simulink model "B34SNSTest"  (R2023b)
settings: Solver=VariableStepAuto  StartTime=0.0  StopTime=100  RelTol=1E-4  AbsTol=1E-4
values from neighbouring files (symbols this model uses):
  AinfKA_h_B34 = -60    [B34.m]    (also in CtrlParaSNSTuning.m)
  AinfKA_p_B34 = 1.0    (= 1)    [B34.m]    (also in CtrlParaSNSTuning.m)
  AinfKA_s_B34 = 1.0    (= 1)    [B34.m]    (also in CtrlParaSNSTuning.m)
  AKA_B34_0 = 0.4    [B34.m]    (also in CtrlParaSNSTuning.m; InitPara.m)
  BinfKA_h_B34 = -55.0    (= -55)    [B34.m]    (also in CtrlParaSNSTuning.m)
  BinfKA_p_B34 = 2.0    (= 2)    [B34.m]    (also in CtrlParaSNSTuning.m)
  BinfKA_s_B34 = 1.0    (= 1)    [B34.m]    (also in CtrlParaSNSTuning.m)
  BKA_B34_0 = 0.4    [B34.m]    (also in CtrlParaSNSTuning.m; InitPara.m)
  Cm_B34 = 0.01    [B34.m]    (also in CtrlParaSNSTuning.m)
  EKA_B34 = -60    [B34.m]    (also in CtrlParaSNSTuning.m)
  EL_B34 = -60    [B34.m]    (also in CtrlParaSNSTuning.m)
  gKA_B34 = 1.25    [B34.m]    (also in CtrlParaSNSTuning.m)
  gL_B34 = 0.1    [B34.m]    (also in CtrlParaSNSTuning.m)
  pKA_B34 = 2    [B34.m]    (also in CtrlParaSNSTuning.m)
  RKA_B34 = 0    [B34.m]    (also in CtrlParaSNSTuning.m)
  RL_B34 = 0    [B34.m]    (also in CtrlParaSNSTuning.m)
  tAKA_h_B34 = -56    [B34.m]    (also in CtrlParaSNSTuning.m)
  tAKA_p_B34 = 2.0    (= 2)    [B34.m]    (also in CtrlParaSNSTuning.m)
  tAKA_s_B34 = 1.0    (= 1)    [B34.m]    (also in CtrlParaSNSTuning.m)
  tAKA_tmax_B34 = 0.2    [B34.m]    (also in CtrlParaSNSTuning.m)
  tAKA_tmin_B34 = 0.02    [B34.m]    (also in CtrlParaSNSTuning.m)
  tBKA_tmax_B34 = 0.5    [B34.m]    (also in CtrlParaSNSTuning.m)
  V_B34_0 = -60    [B34.m]    (also in CtrlParaSNSTuning.m; InitPara.m)
  V_max = 130/3    (= 43.3333333333)    [B34.m]    (also in B4.m; CtrlParaSNSTuning.m)
  V_min = 3.2/3    (= 1.06666666667)    [B34.m]    (also in B4.m = 5; CtrlParaSNSTuning.m = 5)
undefined symbols (not defined in the file or in its folder): Iapp
settings Model: SimulationMode=accelerator  Creator=liyan  LastModifiedBy=Yanjun
settings ModelReferenceCC: EnableRefExpFcnMdlSchedulingChecks=on

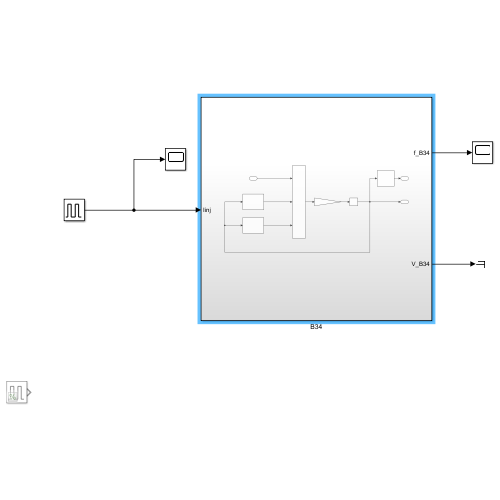
[thumbnail: Simulink's stored preview of the top-level diagram]
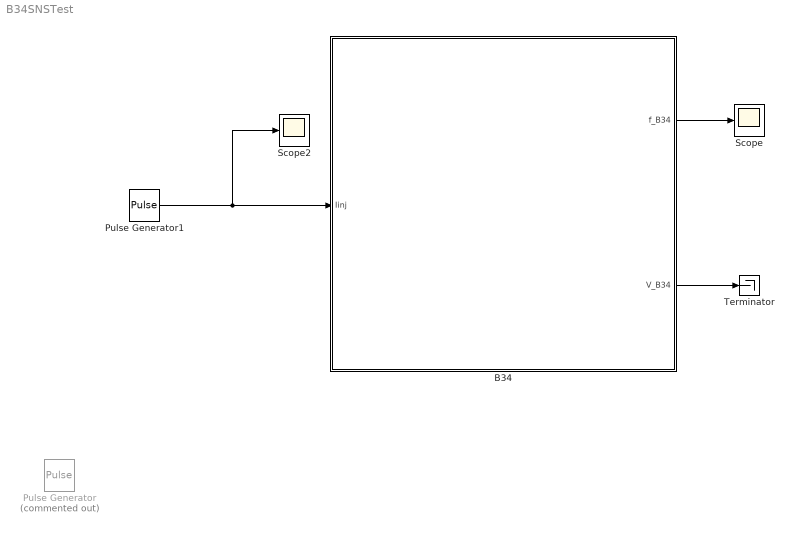
== system B34SNSTest ==
  B34 : Subsystem
      settings: PortSchema="{\"entries\":[{\"content\":{\"sides\":[{\"content\":{\"connectorIds\":[]},\"type\":\"ConnectorPlacement.EquallySpacedRectSide\",\"uuid\":\"791cb9f9-6115-440d-b81f-06b3e1381d11\"},{\"content\":{\"connectorIds\":[],\"side\":\"RIGHT\"},\"type\":\"ConnectorPlacement.EquallySpacedRectSide\",\"uuid\":\"7c3ff3b3-a19c-4513-b6da-d54d5819647a\"},{\"content\":{\"connectorIds\":[\"Out1\",\"Out2\"],\"side\":\"TOP\"},\"type\":\"ConnectorPlacement.EquallySpacedRectSide\",\"uuid\":\"74d2471c-8ad6-4c64-9275-9831c9b942a4\"},{\"content\":{\"connectorIds\":[\"In1\"],\"side\":\"BOTTOM\"},\"type\":\"ConnectorPlacement.EquallySpacedRectSide\",\"uuid\":\"d13eda8e-856d-496c-9126-6826d7a5e8e6\"}]},\"type\":\"ConnectorPlacement.EquallySpacedConnector\",\"uuid\":\"cfc5e95a-0097-4eeb-afba-0bc23a3dc93b\"}],\"packageUris\":[\"http://schema.mathworks.com/mf0/Connector/R2020b\"],\"version\":\"1.0\"}"
  Pulse Generator : DiscretePulseGenerator  Commented=on  PulseType=Time based  Amplitude=Iapp  Period=30  PulseWidth=10/30*100  PhaseDelay=10
  Pulse Generator1 : DiscretePulseGenerator  PulseType=Time based  Amplitude=Iapp  Period=100  PulseWidth=10/100*100  PhaseDelay=35
  Scope : Scope
  Scope2 : Scope
  Terminator : Terminator
  wires:
  Pulse Generator1/1 -> B34/1(Iinj), Scope2/1
  B34/2(f_B34) -> Scope/1
  B34/1(V_B34) -> Terminator/1

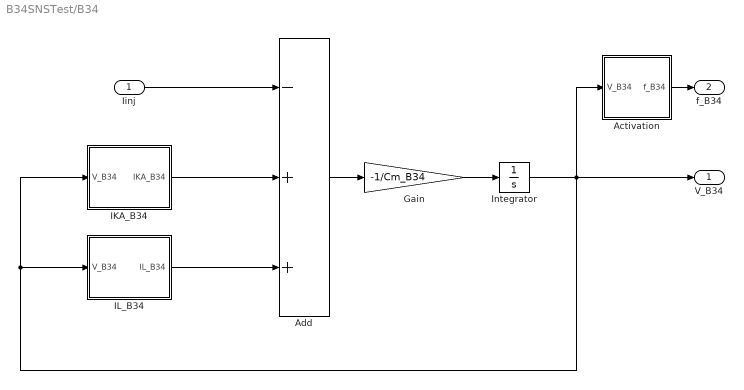
== system B34SNSTest/B34 ==
  Iinj : Inport
  Activation : Subsystem
  Add : Sum  Inputs=-++
  Gain : Gain  Gain=-1/Cm_B34
  IKA_B34 : Subsystem
  IL_B34 : Subsystem
  Integrator : Integrator  InitialCondition=V_B34_0
  V_B34 : Outport
  f_B34 : Outport  Port=2
  wires:
  Gain/1 -> Integrator/1
  Add/1 -> Gain/1
  Activation/1(f_B34) -> f_B34/1
  IL_B34/1(IL_B34) -> Add/3
  Integrator/1 -> Activation/1(V_B34), IKA_B34/1(V_B34), IL_B34/1(V_B34), V_B34/1
  Iinj/1 -> Add/1
  IKA_B34/1(IKA_B34) -> Add/2

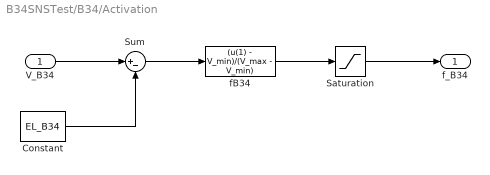
== system B34SNSTest/B34/Activation ==
  V_B34 : Inport
  Constant : Constant  Value=EL_B34
  Saturation : Saturate  UpperLimit=1  LowerLimit=0
  Sum : Sum  Inputs=|+-
  fB34 : MATLABFcn  MATLABFcn=(u(1) - V_min)/(V_max - V_min)
  f_B34 : Outport
  wires:
  fB34/1 -> Saturation/1
  Saturation/1 -> f_B34/1
  Sum/1 -> fB34/1
  V_B34/1 -> Sum/1
  Constant/1 -> Sum/2

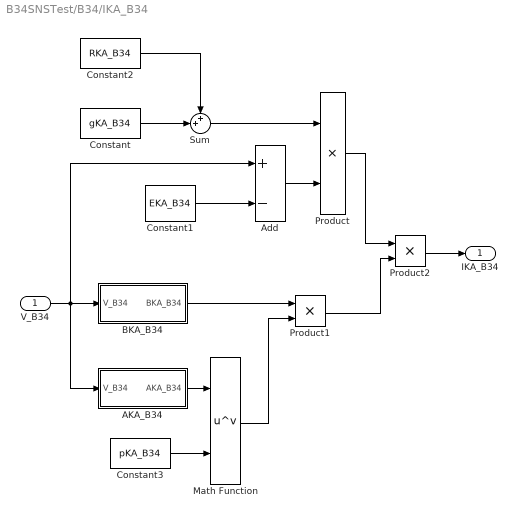
== system B34SNSTest/B34/IKA_B34 ==
  V_B34 : Inport
  AKA_B34 : Subsystem
  Add : Sum  Inputs=+-
  BKA_B34 : Subsystem
  Constant : Constant  Value=gKA_B34
  Constant1 : Constant  Value=EKA_B34
  Constant2 : Constant  Value=RKA_B34
  Constant3 : Constant  Value=pKA_B34
  Math Function : Math  Operator=pow
  Product : Product
  Product1 : Product
  Product2 : Product
  Sum : Sum  Inputs=++|
  IKA_B34 : Outport
  wires:
  Add/1 -> Product/2
  Constant1/1 -> Add/2
  V_B34/1 -> AKA_B34/1(V_B34), BKA_B34/1(V_B34), Add/1
  Product/1 -> Product2/1
  Product1/1 -> Product2/2
  Product2/1 -> IKA_B34/1
  Constant/1 -> Sum/2
  Sum/1 -> Product/1
  Constant2/1 -> Sum/1
  AKA_B34/1(AKA_B34) -> Math Function/1
  Constant3/1 -> Math Function/2
  BKA_B34/1(BKA_B34) -> Product1/1
  Math Function/1 -> Product1/2

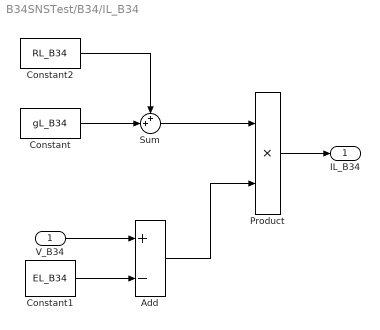
== system B34SNSTest/B34/IL_B34 ==
  V_B34 : Inport
  Add : Sum  Inputs=+-
  Constant : Constant  Value=gL_B34
  Constant1 : Constant  Value=EL_B34
  Constant2 : Constant  Value=RL_B34
  Product : Product
  Sum : Sum  Inputs=++|
  IL_B34 : Outport
  wires:
  Constant1/1 -> Add/2
  V_B34/1 -> Add/1
  Constant2/1 -> Sum/1
  Sum/1 -> Product/1
  Constant/1 -> Sum/2
  Add/1 -> Product/2
  Product/1 -> IL_B34/1

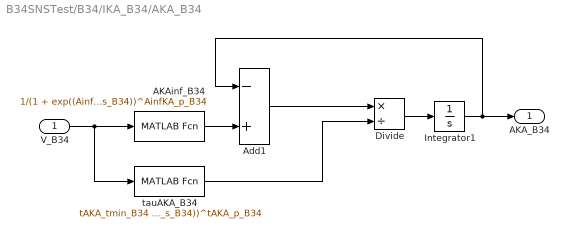
== system B34SNSTest/B34/IKA_B34/AKA_B34 ==
  V_B34 : Inport
  AKAinf_B34 : MATLABFcn  MATLABFcn=1/(1 + exp((AinfKA_h_B34 - u(1))/AinfKA_s_B34))^AinfKA_p_B34
  Add1 : Sum  Inputs=-+
  Divide : Product  Inputs=*/
  Integrator1 : Integrator  InitialCondition=AKA_B34_0
  tauAKA_B34 : MATLABFcn  MATLABFcn=tAKA_tmin_B34 + (tAKA_tmax_B34 - tAKA_tmin_B34)/(1 + exp((u(1) - tAKA_h_B34)/tAKA_s_B34))^tAKA_p_B34
  AKA_B34 : Outport
  wires:
  tauAKA_B34/1 -> Divide/2
  Divide/1 -> Integrator1/1
  V_B34/1 -> tauAKA_B34/1, AKAinf_B34/1
  Integrator1/1 -> Add1/1, AKA_B34/1
  Add1/1 -> Divide/1
  AKAinf_B34/1 -> Add1/2

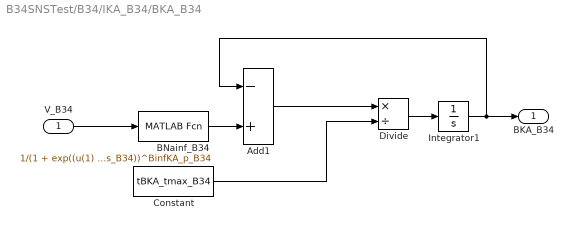
== system B34SNSTest/B34/IKA_B34/BKA_B34 ==
  V_B34 : Inport
  Add1 : Sum  Inputs=-+
  BNainf_B34 : MATLABFcn  MATLABFcn=1/(1 + exp((u(1) - BinfKA_h_B34)/BinfKA_s_B34))^BinfKA_p_B34
  Constant : Constant  Value=tBKA_tmax_B34
  Divide : Product  Inputs=*/
  Integrator1 : Integrator  InitialCondition=BKA_B34_0
  BKA_B34 : Outport
  wires:
  Constant/1 -> Divide/2
  Divide/1 -> Integrator1/1
  V_B34/1 -> BNainf_B34/1
  Integrator1/1 -> Add1/1, BKA_B34/1
  Add1/1 -> Divide/1
  BNainf_B34/1 -> Add1/2
